simulink model "RTinductionmotorNov28new"  (R2017b)
settings: Solver=VariableStepAuto  StartTime=0.0  StopTime=0.25  MaxStep=0.0000001  RelTol=1e-3
undefined symbols (not defined in the file or in its folder): biasA, biasB, f
settings Model: Creator=adam_  LastModifiedBy=Yaipiti
settings DataIOCC: ReturnWorkspaceOutputs=on
settings SFSimCC: SimUseLocalCustomCode=on
settings RTWCC: RTWUseLocalCustomCode=on

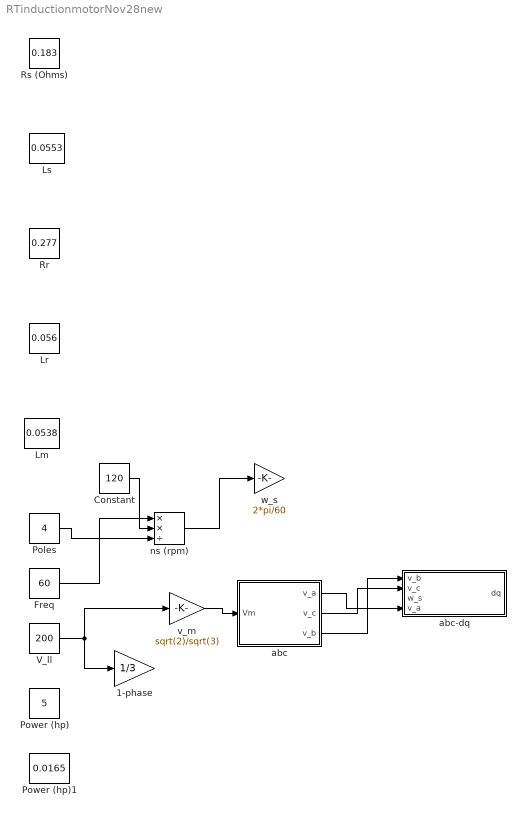
== system RTinductionmotorNov28new ==
  1-phase : Gain  Gain=1/3
  Constant : Constant  Value=120
  Freq : Constant  Value=60
  "Lm " : Constant  Value=0.0538
  Lr : Constant  Value=0.056
  "Ls " : Constant  Value=0.0553
  Poles : Constant  Value=4
  Power (hp) : Constant  Value=5
  Power (hp)1 : Constant  Value=0.0165
  "Rr " : Constant  Value=0.277
  Rs (Ohms) : Constant  Value=0.183
  V_ll : Constant  Value=200
  abc : Subsystem
  abc-dq : Subsystem
  ns (rpm) : Product  Inputs=**/
  v_m : Gain  Gain=sqrt(2)/sqrt(3)
  w_s : Gain  Gain=2*pi/60
  wires:
  V_ll/1 -> v_m/1, 1-phase/1
  Freq/1 -> ns (rpm)/1
  Poles/1 -> ns (rpm)/3
  Constant/1 -> ns (rpm)/2
  ns (rpm)/1 -> w_s/1
  v_m/1 -> abc/1(Vm)
  abc/1(v_a) -> abc-dq/4(v_a)
  abc/2(v_c) -> abc-dq/2(v_c)
  abc/3(v_b) -> abc-dq/1(v_b)

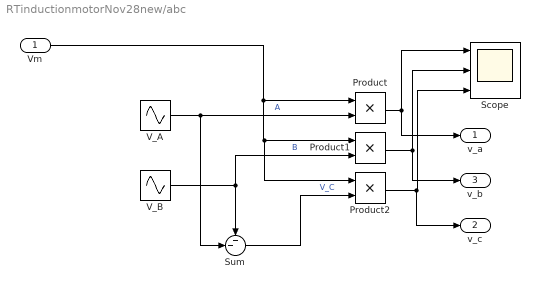
== system RTinductionmotorNov28new/abc ==
  Vm : Inport
  Product : Product
  Product1 : Product
  Product2 : Product
  Scope : Scope  NumInputPorts=3
  Sum : Sum  Inputs=--|  InputSameDT=on  SaturateOnIntegerOverflow=on  OutDataTypeStr=Inherit: Same as first input
  V_A : Sin  Bias=biasA  Frequency=2*pi*f  Phase=pi/2  SampleTime=0
  V_B : Sin  Bias=biasB  Frequency=2*pi*f  Phase=-pi/6  SampleTime=0
  v_a : Outport
  v_c : Outport  Port=2
  v_b : Outport  Port=3
  wires:
  Vm/1 -> Product2/1, Product1/1, Product/1
  Sum/1 -> Product2/2  "V_C"
  V_A/1 -> Product/2, Sum/2  "A"
  V_B/1 -> Product1/2, Sum/1  "B"
  Product/1 -> Scope/1, v_a/1
  Product1/1 -> Scope/2, v_b/1
  Product2/1 -> v_c/1, Scope/3

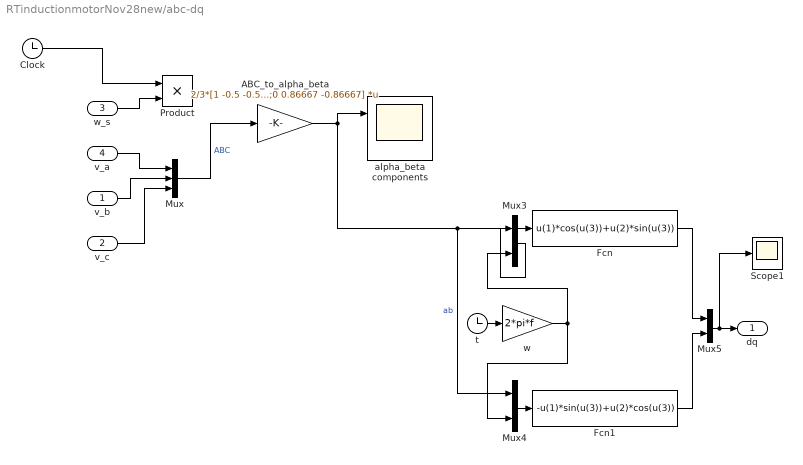
== system RTinductionmotorNov28new/abc-dq ==
  v_b : Inport
  v_c : Inport  Port=2
  w_s : Inport  Port=3
  v_a : Inport  Port=4
  ABC_to_alpha_beta : Gain  Gain=2/3*[1 -0.5 -0.5;0 0.86667 -0.86667]  Multiplication=Matrix(K*u)  SaturateOnIntegerOverflow=on  OutDataTypeStr=Inherit: Same as input  ParamDataTypeStr=Inherit: Same as input
  Clock : Clock
  Fcn : Fcn  Expr=u(1)*cos(u(3))+u(2)*sin(u(3))
  Fcn1 : Fcn  Expr=-u(1)*sin(u(3))+u(2)*cos(u(3))
  Mux : Mux  Inputs=3
  Mux3 : Mux  Inputs=2
  Mux4 : Mux  Inputs=2
  Mux5 : Mux  Inputs=2
  Product : Product
  Scope1 : Scope
  alpha_beta components : Scope  NumInputPorts=2
  t : Clock
  w : Gain  Gain=2*pi*f  SaturateOnIntegerOverflow=on  OutDataTypeStr=Inherit: Same as input  ParamDataTypeStr=Inherit: Same as input
  dq : Outport
  wires:
  Mux/1 -> ABC_to_alpha_beta/1  "ABC"
  ABC_to_alpha_beta/1 -> Mux4/1, Mux3/1, alpha_beta components/1  "ab"
  v_a/1 -> Mux/1
  v_b/1 -> Mux/2
  v_c/1 -> Mux/3
  Clock/1 -> Product/1
  w_s/1 -> Product/2
  Fcn1/1 -> Mux5/2
  Fcn/1 -> Mux5/1
  w/1 -> Mux3/2, Mux4/2
  Mux3/1 -> Fcn/1
  Mux5/1 -> Scope1/1, dq/1
  Mux4/1 -> Fcn1/1
  t/1 -> w/1
